simulink model "Simulacion_stepper_2024a"  (R2024a)
settings: Solver=ode4  StartTime=0.0  StopTime=Time_simulation  FixedStep=1/frecuency_simulation  RelTol=1e-3
InitFcn:
  | %%InitFcn();
StopFcn:
  | %%FinishFcn
model workspace (MAT data in the model file):
  Ts_stepper = 0.001
values from neighbouring files (symbols this model uses):
  B = motor_params.B_internal    [bode.m]    (also in current_observer.m = 0.0005; discretizacion.m = [ 1/L, 0; ekf_4_estados.m = params.B; obs_ctrl_back_emf_ext.m = [1/L 0)
  B0 = 3*wn_w - BJ_hat    [Barrido_B.m]    (also in Barrido_J.m; InitFcn.m = 449.962302294)
  B1 = 3*wn_w^2 - B0*BJ_hat    [Barrido_B.m]    (also in Barrido_J.m; InitFcn.m = 64448.3670019)
  B2 = -(J_var/P)*(wn_w^3)    [Barrido_B.m]    (also in Barrido_J.m; InitFcn.m = -0.364323750994)
  B_internal = 1e-4    (= 0.0001)    [InitFcn.m]
  B_var = B_internal* B_factors(k)    [Barrido_B.m]    (also in Barrido_J.m = B_real; InitFcn.m = 0.0001)
  frecuency_simulation = 10e3    (= 10000)    [InitFcn.m]
  I_nom = 1    [InitFcn.m]    (also in salient_motor.m)
  J = motor_params.J_internal    [bode.m]    (also in current_observer.m = 0.008; ekf_4_estados.m = params.J; obs_ctrl_back_emf_ext.m = 0.008; obs_y_contrl_back_emd.m = 0.008)
  J_internal = 4.7/1000000    (= 4.7e-06)    [InitFcn.m]
  J_var = J_real    [Barrido_B.m]    (also in Barrido_J.m = J_internal * J_factors(k); InitFcn.m = 4.7e-06)
  Ke = Kt    [InitFcn.m]    (also in current_observer.m = 0.0055; ekf_4_estados.m = params.Ke; observer.m = Pvec(3); salient_motor.m = 0.0066)
  Ki_d = wd_d*R    (= 3926.99081699)    [InitFcn.m]    (also in bode.m = PI_dq_params.Ki_d_salient)
  Ki_d_salient = wd_d^2*Ld    (= 21491.0635834)    [InitFcn.m]
  Ki_q = wd_q*R    (= 3926.99081699)    [InitFcn.m]    (also in bode.m = PI_dq_params.Ki_q_salient)
  Ki_q_salient = wd_q^2*Lq    (= 7846.33549887)    [InitFcn.m]
  Ki_w = (wn_w^2)*J_var/Kt    [Barrido_B.m]    (also in Barrido_J.m; InitFcn.m; bode.m = PI_MTPA_params.Ki_w)
  Kp_d = wd_d*L    (= 9.42477796077)    [InitFcn.m]    (also in bode.m = PI_dq_params.Kp_d_salient)
  Kp_d_salient = 2*shi_d*wd_d*Ld -R    (= 16.845833313)    [InitFcn.m]
  Kp_q = wd_q*L    (= 9.42477796077)    [InitFcn.m]    (also in bode.m = PI_dq_params.Kp_q_salient)
  Kp_q_salient = 2*shi_q*wd_q*Lq-R    (= 4.56311709936)    [InitFcn.m]
  Kp_w = (2*shi_w*wn_w*J_var)/Kt    [Barrido_B.m]    (also in Barrido_J.m; InitFcn.m; bode.m = PI_MTPA_params.Kp_w)
  Kt = Thold / (sqrt(2) * I_nom)    [InitFcn.m]    (also in current_observer.m = 0.275; ekf_4_estados.m = params.Kt; frecuencia_max.m = 0.33; observer.m = Pvec(4))
  L = 6/1000    (= 0.006)    [InitFcn.m]    (also in current_observer.m = place(A', C', 10*eig(A)).'; desfase.m = lags(k); discretizacion.m = 0.01; frecuencia_max.m)
  Ld = L0 + L2    [Copy_of_PMSM_salient.m]    (also in InitFcn.m = 0.00871; bode.m = motor_params.Ld; ekf_4_estados.m = params.Ld; salient_motor.m = 0.00871)
  Lq = L0 - L2    [Copy_of_PMSM_salient.m]    (also in InitFcn.m = 0.00318; bode.m = motor_params.Lq; ekf_4_estados.m = params.Lq; salient_motor.m = 0.00318)
  N_steps = 360/Step_angle    (= 200)    [InitFcn.m]
  P = N_teeths/2    (= 50)    [InitFcn.m]    (also in bode.m = motor_params.P; ekf_4_estados.m = P_pred; frecuencia_max.m; salient_motor.m)
  Phi = pi/2    (= 1.57079632679)    [InitFcn.m]    (also in ekf_4_estados.m = eye(4) + Ts_eff*A)
  Psi = Kt/P    [InitFcn.m]    (also in bode.m = motor_params.Ke; salient_motor.m = 0.0066)
  R = 2.5    [InitFcn.m]    (also in bode.m = motor_params.R; current_observer.m = 3.4; discretizacion.m = 3.4; ekf_4_estados.m = params.R)
  sample_time = 1/frecuency_simulation    (= 0.0001)    [InitFcn.m]
  Tdm = 18/1000    (= 0.018)    [InitFcn.m]    (also in salient_motor.m)
  Ts_current = 1/f_current    (= 0.0001)    [InitFcn.m]
  Ts_DO = Ts_Wm    (= 0.0001)    [InitFcn.m]
  Ts_ekf = 1/f_ekf    (= 0.0001)    [InitFcn.m]
  Ts_Wm = Ts_current    (= 0.0001)    [InitFcn.m]
  Vdc = 12    [InitFcn.m]    (also in frecuencia_max.m)
undefined symbols (not defined in the file or in its folder): DiscIntNeverNeededParam
libraries: fl_lib x27, nesl_utility x19, spsMosfetLib x16, simulink x8, eeTransforms x4, spsDCVoltageSourceLib x4, spsVoltageMeasurementLib x4, ee_lib x3, slexportprevious_tp74def212_4eb8_4616_a2bc_f4e795655e99 x1, spsTriangleGeneratorLib x1, spspowerguiLib x1
(part 3 of 4)

== system Simulacion_stepper_2024a/Triggered Subsystem8 ==
  Wm_ref : Inport
  Wm : Inport  Port=2
  Tl_Tdm : Inport  Port=3
  function : TriggerPort  TriggerType=function-call  VariantControl=(inherit)  SampleTime=1/100
  C/C++ Code Block : S-Function  Commented=on  FunctionName=PI_dq  SFunctionModules=PI_dq_wrapper.c  SFunctionDeploymentMode=off  EnableBusSupport=off  mask(S-Function Builder){}
      mask help: Simulink:masks:SFunctionBuilder_MD
      mask init: same as Simulacion_stepper_2024a/Triggered Subsystem1/C/C++ Code Block1
      settings: CopyFcn=set_param(gcbh,'LinkStatus','none')  OpenFcn=sfunctionwizard(gcbh)
      mask Display:
      | plot(val(:,1),val(:,2))
      | disp(sys)
      | port_label('input',1,sprintf('%s', 'Ia'),'interpreter','tex')
      | port_label('input',2,sprintf('%s', 'Ib'),'interpreter','tex')
      | port_label('input',3,sprintf('%s', 'Wm\_ref'),'interpreter','tex')
      | port_label('input',4,sprintf('%s', 'Wm\_ext'),'interpreter','tex')
      | port_label('input',5,sprintf('%s', 'Kp\_current'),'interpreter','tex')
      | port_label('input',6,sprintf('%s', 'Ki\_current'),'interpreter','tex')
      | port_label('input',7,sprintf('%s', 'Kd\_current'),'interpreter','tex')
      | port_label('input',8,sprintf('%s', 'sample\_time\_ext'),'interpreter','tex')
      | port_label('input',9,sprintf('%s', 'Vdc\_ext'),'interpreter','tex')
      | port_label('input',10,sprintf('%s', 'R\_ext'),'interpreter','tex')
      | port_label('input',11,sprintf('%s', 'Ld\_ext'),'interpreter','tex')
      | port_label('input',12,sprintf('%s', 'Lq\_ext'),'interpreter','tex')
      | port_label('input',13,sprintf('%s', 'Ke\_ext'),'interpreter','tex')
      | port_label('input',14,sprintf('%s', 'Theta\_ext'),'interpreter','tex')
      | port_label('input',15,sprintf('%s', 'Kp\_wm'),'interpreter','tex')
      | port_label('input',16,sprintf('%s', 'Ki\_wm'),'interpreter','tex')
      | port_label('input',17,sprintf('%s', 'Tl\_Tdm'),'interpreter','tex')
      | port_label('input',18,sprintf('%s', 'B'),'interpreter','tex')
      | port_label('input',19,sprintf('%s', 'Kt\_ext'),'interpreter','tex')
      | port_label('output',1,sprintf('%s', 'Ud'),'interpreter','tex')
      | port_label('output',2,sprintf('%s', 'Uq'),'interpreter','tex')
      | port_label('output',3,sprintf('%s', 'Id'),'interpreter','tex')
      | port_label('output',4,sprintf('%s', 'Iq'),'interpreter','tex')
      | port_label('output',5,sprintf('%s', 'Iq\_ref\_aux'),'interpreter','tex')
  Constant : Constant  Value=B_var  OutDataTypeStr=double
  Constant1 : Constant  Value=Kp_w  OutDataTypeStr=double
  Constant11 : Constant  Value=Ki_w  OutDataTypeStr=double
  Constant12 : Constant  Value=Kt  OutDataTypeStr=double
  Constant2 : Constant  Value=I_nom  OutDataTypeStr=double
  Constant3 : Constant  Value=Ts_Wm  OutDataTypeStr=double
  MATLAB Function : MATLAB Function  TreatAsAtomicUnit=on
  Iq_ref : Outport
  wires:
  MATLAB Function/1(Iq_ref) -> Iq_ref/1
  Wm_ref/1 -> MATLAB Function/1(Wm_ref)
  Wm/1 -> MATLAB Function/2(Wm)
  Constant12/1 -> MATLAB Function/8(Kt)
  Constant/1 -> MATLAB Function/7(B)
  Tl_Tdm/1 -> MATLAB Function/6(Tl_tdm)
  Constant1/1 -> MATLAB Function/4(Kp_w)
  Constant11/1 -> MATLAB Function/5(Ki_w)
  Constant3/1 -> MATLAB Function/3(Ts)
  Constant2/1 -> MATLAB Function/9(Imax)

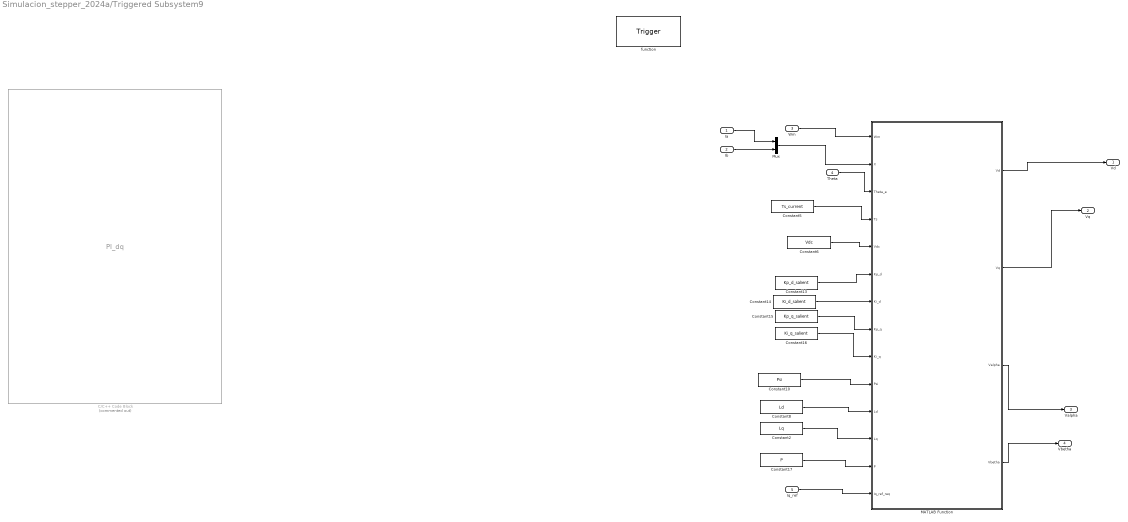
== system Simulacion_stepper_2024a/Triggered Subsystem9 ==
  Ia : Inport
  Ib : Inport  Port=2
  Wm : Inport  Port=3
  Theta : Inport  Port=4
  Iq_ref : Inport  Port=5
  function : TriggerPort  TriggerType=function-call  VariantControl=(inherit)  SampleTime=1/100
  C/C++ Code Block : S-Function  Commented=on  FunctionName=PI_dq  SFunctionModules=PI_dq_wrapper.c  SFunctionDeploymentMode=off  EnableBusSupport=off  mask(S-Function Builder){}
      mask help: Simulink:masks:SFunctionBuilder_MD
      mask init: same as Simulacion_stepper_2024a/Triggered Subsystem1/C/C++ Code Block1
      settings: CopyFcn=set_param(gcbh,'LinkStatus','none')  OpenFcn=sfunctionwizard(gcbh)
      mask Display:
      | plot(val(:,1),val(:,2))
      | disp(sys)
      | port_label('input',1,sprintf('%s', 'Ia'),'interpreter','tex')
      | port_label('input',2,sprintf('%s', 'Ib'),'interpreter','tex')
      | port_label('input',3,sprintf('%s', 'Wm\_ref'),'interpreter','tex')
      | port_label('input',4,sprintf('%s', 'Wm\_ext'),'interpreter','tex')
      | port_label('input',5,sprintf('%s', 'Kp\_current'),'interpreter','tex')
      | port_label('input',6,sprintf('%s', 'Ki\_current'),'interpreter','tex')
      | port_label('input',7,sprintf('%s', 'Kd\_current'),'interpreter','tex')
      | port_label('input',8,sprintf('%s', 'sample\_time\_ext'),'interpreter','tex')
      | port_label('input',9,sprintf('%s', 'Vdc\_ext'),'interpreter','tex')
      | port_label('input',10,sprintf('%s', 'R\_ext'),'interpreter','tex')
      | port_label('input',11,sprintf('%s', 'Ld\_ext'),'interpreter','tex')
      | port_label('input',12,sprintf('%s', 'Lq\_ext'),'interpreter','tex')
      | port_label('input',13,sprintf('%s', 'Ke\_ext'),'interpreter','tex')
      | port_label('input',14,sprintf('%s', 'Theta\_ext'),'interpreter','tex')
      | port_label('input',15,sprintf('%s', 'Kp\_wm'),'interpreter','tex')
      | port_label('input',16,sprintf('%s', 'Ki\_wm'),'interpreter','tex')
      | port_label('input',17,sprintf('%s', 'Tl\_Tdm'),'interpreter','tex')
      | port_label('input',18,sprintf('%s', 'B'),'interpreter','tex')
      | port_label('input',19,sprintf('%s', 'Kt\_ext'),'interpreter','tex')
      | port_label('output',1,sprintf('%s', 'Ud'),'interpreter','tex')
      | port_label('output',2,sprintf('%s', 'Uq'),'interpreter','tex')
      | port_label('output',3,sprintf('%s', 'Id'),'interpreter','tex')
      | port_label('output',4,sprintf('%s', 'Iq'),'interpreter','tex')
      | port_label('output',5,sprintf('%s', 'Iq\_ref\_aux'),'interpreter','tex')
  Constant10 : Constant  Value=Psi  OutDataTypeStr=double
  Constant13 : Constant  Value=Kp_d_salient  OutDataTypeStr=double
  Constant14 : Constant  Value=Ki_d_salient  OutDataTypeStr=double
  Constant15 : Constant  Value=Kp_q_salient  OutDataTypeStr=double
  Constant16 : Constant  Value=Ki_q_salient  OutDataTypeStr=double
  Constant17 : Constant  Value=P  OutDataTypeStr=double
  Constant2 : Constant  Value=Lq  OutDataTypeStr=double
  Constant5 : Constant  Value=Ts_current  OutDataTypeStr=double
  Constant6 : Constant  Value=Vdc  OutDataTypeStr=double
  Constant8 : Constant  Value=Ld  OutDataTypeStr=double
  MATLAB Function : MATLAB Function  TreatAsAtomicUnit=on
  Mux : Mux  Inputs=2
  Vd : Outport
  Vq : Outport  Port=2
  Valpha : Outport  Port=3
  Vbetha : Outport  Port=4
  wires:
  MATLAB Function/1(Vd) -> Vd/1
  Wm/1 -> MATLAB Function/1(Wm)
  Ia/1 -> Mux/1
  Ib/1 -> Mux/2
  Mux/1 -> MATLAB Function/2(X)
  Theta/1 -> MATLAB Function/3(Theta_e)
  Constant5/1 -> MATLAB Function/4(Ts)
  Constant6/1 -> MATLAB Function/5(Vdc)
  Constant13/1 -> MATLAB Function/6(Kp_d)
  Constant14/1 -> MATLAB Function/7(Ki_d)
  Constant15/1 -> MATLAB Function/8(Kp_q)
  Constant16/1 -> MATLAB Function/9(Ki_q)
  Constant10/1 -> MATLAB Function/10(Psi)
  Constant8/1 -> MATLAB Function/11(Ld)
  Constant17/1 -> MATLAB Function/13(P)
  Constant2/1 -> MATLAB Function/12(Lq)
  MATLAB Function/2(Vq) -> Vq/1
  Iq_ref/1 -> MATLAB Function/14(Iq_ref_req)
  MATLAB Function/3(Valpha) -> Valpha/1
  MATLAB Function/4(Vbetha) -> Vbetha/1

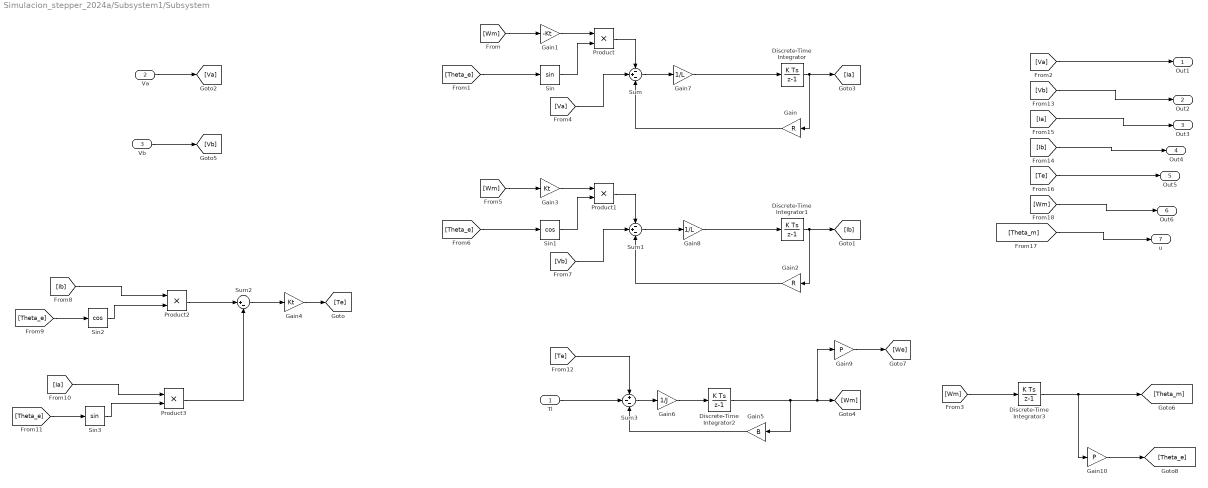
== system Simulacion_stepper_2024a/Subsystem1/Subsystem ==
  Tl : Inport
  Va : Inport  Port=2
  Vb : Inport  Port=3
  Discrete-Time Integrator{,1..3} (4 alike) : DiscreteIntegrator  SampleTime=sample_time  ICPrevOutput=DiscIntNeverNeededParam  ICPrevScaledInput=DiscIntNeverNeededParam
  Gain : Gain  Gain=R
  Gain1 : Gain  Gain=-Kt
  Gain10 : Gain  Gain=P
  Gain2 : Gain  Gain=R
  Gain3 : Gain  Gain=Kt
  Gain4 : Gain  Gain=Kt
  Gain5 : Gain  Gain=B
  Gain6 : Gain  Gain=1/J
  Gain7 : Gain  Gain=1/L
  Gain8 : Gain  Gain=1/L
  Gain9 : Gain  Gain=P
  Product{,1..3} (4 alike) : Product
  Sin : Trigonometry
  Sin1 : Trigonometry  Operator=cos
  Sin2 : Trigonometry  Operator=cos
  Sin3 : Trigonometry
  Sum : Sum  Inputs=-+-
  Sum1 : Sum  Inputs=-+-
  Sum2 : Sum  Inputs=|+-
  Sum3 : Sum  Inputs=+--
  Out1 : Outport
  Out2 : Outport  Port=2
  Out3 : Outport  Port=3
  Out4 : Outport  Port=4
  Out5 : Outport  Port=5
  Out6 : Outport  Port=6
  u : Outport  Port=7
  wires:
  Discrete-Time Integrator/1 -> [Ia], Gain/1
  Discrete-Time Integrator2/1 -> Gain5/1, Gain9/1, [Wm]
  [Wm] -> Discrete-Time Integrator3/1
  [Vb] -> Out2/1
  [Ia] -> Out3/1
  [Ib] -> Out4/1
  [Te] -> Out5/1
  [Wm] -> Out6/1
  [Theta_m] -> u/1
  [Va] -> Out1/1
  Discrete-Time Integrator3/1 -> Gain10/1, [Theta_m]
  Vb/1 -> [Vb]
  Va/1 -> [Va]
  [Wm] -> Gain1/1
  Gain1/1 -> Product/1
  Sin/1 -> Product/2
  [Theta_e] -> Sin/1
  Product/1 -> Sum/1
  [Va] -> Sum/2
  Gain/1 -> Sum/3
  Gain2/1 -> Sum1/3
  [Wm] -> Gain3/1
  [Vb] -> Sum1/2
  [Theta_e] -> Sin1/1
  Gain3/1 -> Product1/1
  Sin1/1 -> Product1/2
  Discrete-Time Integrator1/1 -> [Ib], Gain2/1
  Product1/1 -> Sum1/1
  [Ib] -> Product2/1
  Sin2/1 -> Product2/2
  [Theta_e] -> Sin2/1
  [Ia] -> Product3/1
  [Theta_e] -> Sin3/1
  Sin3/1 -> Product3/2
  Product2/1 -> Sum2/1
  Product3/1 -> Sum2/2
  Sum2/1 -> Gain4/1
  Gain4/1 -> [Te]
  [Te] -> Sum3/1
  Tl/1 -> Sum3/2
  Gain5/1 -> Sum3/3
  Sum3/1 -> Gain6/1
  Sum/1 -> Gain7/1
  Gain7/1 -> Discrete-Time Integrator/1
  Sum1/1 -> Gain8/1
  Gain8/1 -> Discrete-Time Integrator1/1
  Gain6/1 -> Discrete-Time Integrator2/1
  Gain9/1 -> [We]
  Gain10/1 -> [Theta_e]

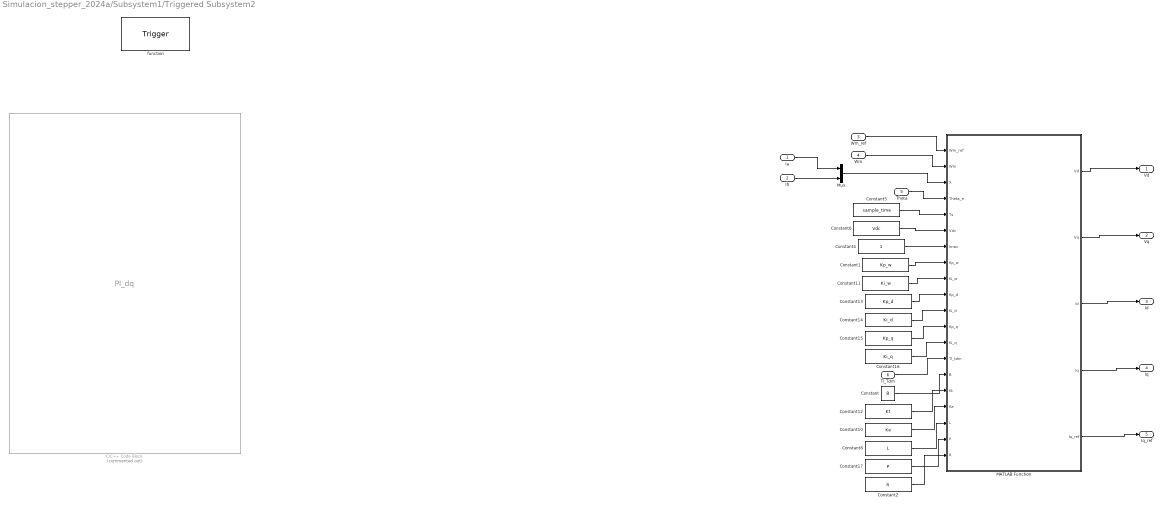
== system Simulacion_stepper_2024a/Subsystem1/Triggered Subsystem2 ==
  Ia : Inport
  Ib : Inport  Port=2
  Wm_ref : Inport  Port=3
  Wm : Inport  Port=4
  Theta : Inport  Port=5
  Tl_Tdm : Inport  Port=6
  function : TriggerPort  TriggerType=function-call  VariantControl=(inherit)  SampleTime=1/100
  C/C++ Code Block : S-Function  Commented=on  FunctionName=PI_dq  SFunctionModules=PI_dq_wrapper.c  SFunctionDeploymentMode=off  EnableBusSupport=off  mask(S-Function Builder){}
      mask help: Simulink:masks:SFunctionBuilder_MD
      mask init: same as Simulacion_stepper_2024a/Triggered Subsystem1/C/C++ Code Block1
      settings: CopyFcn=set_param(gcbh,'LinkStatus','none')  OpenFcn=sfunctionwizard(gcbh)
      mask Display:
      | plot(val(:,1),val(:,2))
      | disp(sys)
      | port_label('input',1,sprintf('%s', 'Ia'),'interpreter','tex')
      | port_label('input',2,sprintf('%s', 'Ib'),'interpreter','tex')
      | port_label('input',3,sprintf('%s', 'Wm\_ref'),'interpreter','tex')
      | port_label('input',4,sprintf('%s', 'Wm\_ext'),'interpreter','tex')
      | port_label('input',5,sprintf('%s', 'Kp\_current'),'interpreter','tex')
      | port_label('input',6,sprintf('%s', 'Ki\_current'),'interpreter','tex')
      | port_label('input',7,sprintf('%s', 'Kd\_current'),'interpreter','tex')
      | port_label('input',8,sprintf('%s', 'sample\_time\_ext'),'interpreter','tex')
      | port_label('input',9,sprintf('%s', 'Vdc\_ext'),'interpreter','tex')
      | port_label('input',10,sprintf('%s', 'R\_ext'),'interpreter','tex')
      | port_label('input',11,sprintf('%s', 'Ld\_ext'),'interpreter','tex')
      | port_label('input',12,sprintf('%s', 'Lq\_ext'),'interpreter','tex')
      | port_label('input',13,sprintf('%s', 'Ke\_ext'),'interpreter','tex')
      | port_label('input',14,sprintf('%s', 'Theta\_ext'),'interpreter','tex')
      | port_label('input',15,sprintf('%s', 'Kp\_wm'),'interpreter','tex')
      | port_label('input',16,sprintf('%s', 'Ki\_wm'),'interpreter','tex')
      | port_label('input',17,sprintf('%s', 'Tl\_Tdm'),'interpreter','tex')
      | port_label('input',18,sprintf('%s', 'B'),'interpreter','tex')
      | port_label('input',19,sprintf('%s', 'Kt\_ext'),'interpreter','tex')
      | port_label('output',1,sprintf('%s', 'Ud'),'interpreter','tex')
      | port_label('output',2,sprintf('%s', 'Uq'),'interpreter','tex')
      | port_label('output',3,sprintf('%s', 'Id'),'interpreter','tex')
      | port_label('output',4,sprintf('%s', 'Iq'),'interpreter','tex')
      | port_label('output',5,sprintf('%s', 'Iq\_ref\_aux'),'interpreter','tex')
  Constant : Constant  Value=B  OutDataTypeStr=double
  Constant1 : Constant  Value=Kp_w  OutDataTypeStr=double
  Constant10 : Constant  Value=Ke  OutDataTypeStr=double
  Constant11 : Constant  Value=Ki_w  OutDataTypeStr=double
  Constant12 : Constant  Value=Kt  OutDataTypeStr=double
  Constant13 : Constant  Value=Kp_d  OutDataTypeStr=double
  Constant14 : Constant  Value=Ki_d  OutDataTypeStr=double
  Constant15 : Constant  Value=Kp_q  OutDataTypeStr=double
  Constant16 : Constant  Value=Ki_q  OutDataTypeStr=double
  Constant17 : Constant  Value=P  OutDataTypeStr=double
  Constant2 : Constant  Value=R  OutDataTypeStr=double
  Constant4 : Constant  OutDataTypeStr=double
  Constant5 : Constant  Value=sample_time  OutDataTypeStr=double
  Constant6 : Constant  Value=Vdc  OutDataTypeStr=double
  Constant8 : Constant  Value=L  OutDataTypeStr=double
  MATLAB Function : MATLAB Function  TreatAsAtomicUnit=on
  Mux : Mux  Inputs=2
  Vd : Outport
  Vq : Outport  Port=2
  Id : Outport  Port=3
  Iq : Outport  Port=4
  Iq_ref : Outport  Port=5
  wires:
  MATLAB Function/1(Vd) -> Vd/1
  MATLAB Function/2(Vq) -> Vq/1
  MATLAB Function/3(Id) -> Id/1
  MATLAB Function/4(Iq) -> Iq/1
  MATLAB Function/5(Iq_ref) -> Iq_ref/1
  Wm_ref/1 -> MATLAB Function/1(Wm_ref)
  Wm/1 -> MATLAB Function/2(Wm)
  Ia/1 -> Mux/1
  Ib/1 -> Mux/2
  Mux/1 -> MATLAB Function/3(X)
  Theta/1 -> MATLAB Function/4(Theta_e)
  Constant5/1 -> MATLAB Function/5(Ts)
  Constant6/1 -> MATLAB Function/6(Vdc)
  Constant12/1 -> MATLAB Function/16(Kt)
  Constant/1 -> MATLAB Function/15(B)
  Tl_Tdm/1 -> MATLAB Function/14(Tl_tdm)
  Constant1/1 -> MATLAB Function/8(Kp_w)
  Constant11/1 -> MATLAB Function/9(Ki_w)
  Constant13/1 -> MATLAB Function/10(Kp_d)
  Constant14/1 -> MATLAB Function/11(Ki_d)
  Constant15/1 -> MATLAB Function/12(Kp_q)
  Constant16/1 -> MATLAB Function/13(Ki_q)
  Constant10/1 -> MATLAB Function/17(Ke)
  Constant8/1 -> MATLAB Function/18(L)
  Constant17/1 -> MATLAB Function/19(P)
  Constant4/1 -> MATLAB Function/7(Imax)
  Constant2/1 -> MATLAB Function/20(R)

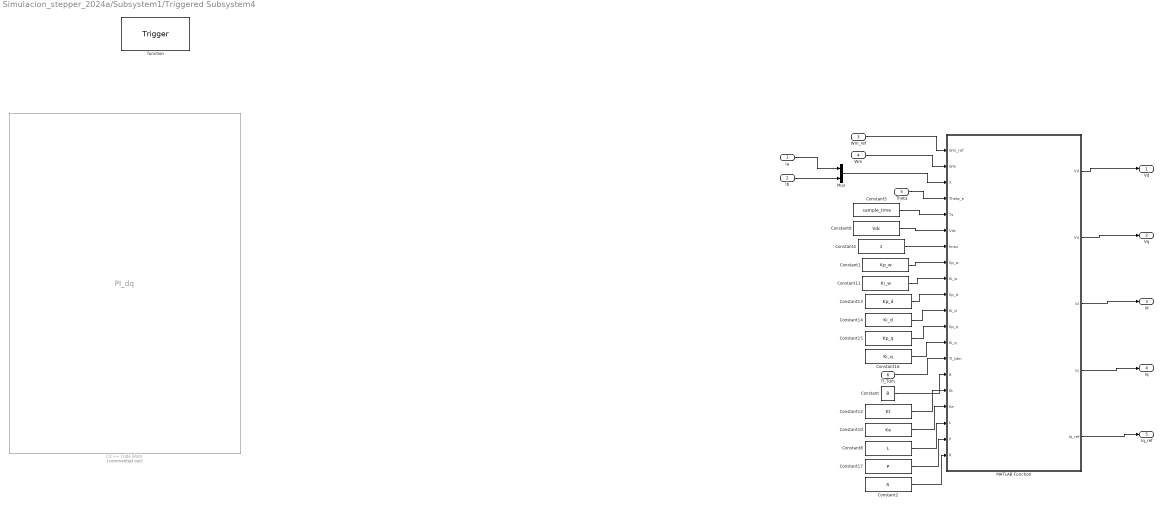
== system Simulacion_stepper_2024a/Subsystem1/Triggered Subsystem4 ==
  Ia : Inport
  Ib : Inport  Port=2
  Wm_ref : Inport  Port=3
  Wm : Inport  Port=4
  Theta : Inport  Port=5
  Tl_Tdm : Inport  Port=6
  function : TriggerPort  TriggerType=function-call  VariantControl=(inherit)  SampleTime=1/100
  C/C++ Code Block : S-Function  Commented=on  FunctionName=PI_dq  SFunctionModules=PI_dq_wrapper.c  SFunctionDeploymentMode=off  EnableBusSupport=off  mask(S-Function Builder){}
      mask help: Simulink:masks:SFunctionBuilder_MD
      mask init: same as Simulacion_stepper_2024a/Triggered Subsystem1/C/C++ Code Block1
      settings: CopyFcn=set_param(gcbh,'LinkStatus','none')  OpenFcn=sfunctionwizard(gcbh)
      mask Display:
      | plot(val(:,1),val(:,2))
      | disp(sys)
      | port_label('input',1,sprintf('%s', 'Ia'),'interpreter','tex')
      | port_label('input',2,sprintf('%s', 'Ib'),'interpreter','tex')
      | port_label('input',3,sprintf('%s', 'Wm\_ref'),'interpreter','tex')
      | port_label('input',4,sprintf('%s', 'Wm\_ext'),'interpreter','tex')
      | port_label('input',5,sprintf('%s', 'Kp\_current'),'interpreter','tex')
      | port_label('input',6,sprintf('%s', 'Ki\_current'),'interpreter','tex')
      | port_label('input',7,sprintf('%s', 'Kd\_current'),'interpreter','tex')
      | port_label('input',8,sprintf('%s', 'sample\_time\_ext'),'interpreter','tex')
      | port_label('input',9,sprintf('%s', 'Vdc\_ext'),'interpreter','tex')
      | port_label('input',10,sprintf('%s', 'R\_ext'),'interpreter','tex')
      | port_label('input',11,sprintf('%s', 'Ld\_ext'),'interpreter','tex')
      | port_label('input',12,sprintf('%s', 'Lq\_ext'),'interpreter','tex')
      | port_label('input',13,sprintf('%s', 'Ke\_ext'),'interpreter','tex')
      | port_label('input',14,sprintf('%s', 'Theta\_ext'),'interpreter','tex')
      | port_label('input',15,sprintf('%s', 'Kp\_wm'),'interpreter','tex')
      | port_label('input',16,sprintf('%s', 'Ki\_wm'),'interpreter','tex')
      | port_label('input',17,sprintf('%s', 'Tl\_Tdm'),'interpreter','tex')
      | port_label('input',18,sprintf('%s', 'B'),'interpreter','tex')
      | port_label('input',19,sprintf('%s', 'Kt\_ext'),'interpreter','tex')
      | port_label('output',1,sprintf('%s', 'Ud'),'interpreter','tex')
      | port_label('output',2,sprintf('%s', 'Uq'),'interpreter','tex')
      | port_label('output',3,sprintf('%s', 'Id'),'interpreter','tex')
      | port_label('output',4,sprintf('%s', 'Iq'),'interpreter','tex')
      | port_label('output',5,sprintf('%s', 'Iq\_ref\_aux'),'interpreter','tex')
  Constant : Constant  Value=B  OutDataTypeStr=double
  Constant1 : Constant  Value=Kp_w  OutDataTypeStr=double
  Constant10 : Constant  Value=Ke  OutDataTypeStr=double
  Constant11 : Constant  Value=Ki_w  OutDataTypeStr=double
  Constant12 : Constant  Value=Kt  OutDataTypeStr=double
  Constant13 : Constant  Value=Kp_d  OutDataTypeStr=double
  Constant14 : Constant  Value=Ki_d  OutDataTypeStr=double
  Constant15 : Constant  Value=Kp_q  OutDataTypeStr=double
  Constant16 : Constant  Value=Ki_q  OutDataTypeStr=double
  Constant17 : Constant  Value=P  OutDataTypeStr=double
  Constant2 : Constant  Value=R  OutDataTypeStr=double
  Constant4 : Constant  OutDataTypeStr=double
  Constant5 : Constant  Value=sample_time  OutDataTypeStr=double
  Constant6 : Constant  Value=Vdc  OutDataTypeStr=double
  Constant8 : Constant  Value=L  OutDataTypeStr=double
  MATLAB Function : MATLAB Function  TreatAsAtomicUnit=on
  Mux : Mux  Inputs=2
  Vd : Outport
  Vq : Outport  Port=2
  Id : Outport  Port=3
  Iq : Outport  Port=4
  Iq_ref : Outport  Port=5
  wires:
  MATLAB Function/1(Vd) -> Vd/1
  MATLAB Function/2(Vq) -> Vq/1
  MATLAB Function/3(Id) -> Id/1
  MATLAB Function/4(Iq) -> Iq/1
  MATLAB Function/5(Iq_ref) -> Iq_ref/1
  Wm_ref/1 -> MATLAB Function/1(Wm_ref)
  Wm/1 -> MATLAB Function/2(Wm)
  Ia/1 -> Mux/1
  Ib/1 -> Mux/2
  Mux/1 -> MATLAB Function/3(X)
  Theta/1 -> MATLAB Function/4(Theta_e)
  Constant5/1 -> MATLAB Function/5(Ts)
  Constant6/1 -> MATLAB Function/6(Vdc)
  Constant12/1 -> MATLAB Function/16(Kt)
  Constant/1 -> MATLAB Function/15(B)
  Tl_Tdm/1 -> MATLAB Function/14(Tl_tdm)
  Constant1/1 -> MATLAB Function/8(Kp_w)
  Constant11/1 -> MATLAB Function/9(Ki_w)
  Constant13/1 -> MATLAB Function/10(Kp_d)
  Constant14/1 -> MATLAB Function/11(Ki_d)
  Constant15/1 -> MATLAB Function/12(Kp_q)
  Constant16/1 -> MATLAB Function/13(Ki_q)
  Constant10/1 -> MATLAB Function/17(Ke)
  Constant8/1 -> MATLAB Function/18(L)
  Constant17/1 -> MATLAB Function/19(P)
  Constant4/1 -> MATLAB Function/7(Imax)
  Constant2/1 -> MATLAB Function/20(R)

== matlab function Simulacion_stepper_2024a/Triggered Subsystem1/MATLAB Function1 ==
  data: U input; x_corr output; X input; Ts input; Kt input; R input; J input; L input; Nr input; B input; Ke input
function x_corr = ekf_5var(U,X,Ts,Kt,R,J,L,Nr,B,Ke)
persistent x_hat P x_pred
%%  x_hat son los estados predichos
%%  x_corr es la salida corregida
%%  P_pre ó Sum_less es la covarianza predicha
%%  P ó sum_more es la covarianza
%%  Rk ó sum_v es la covarianza de incertidumbre del sensor




 %%Iniciamos calculando X_hat[k-1]
 if isempty(x_hat)
     x_hat = zeros(5,1);
     P = diag([1e-4 1e-4 1e-6 1e-10 1e-4]);
     x_corr = zeros(5,1);
     x_pred = zeros(5,1);


 end

Qk = diag([1e-4 1e-4 1e-4 1e-10 1e-6]);
Rk = diag([5e-4 5e-4]);   % ruido de medición

%%1A
%%Predicción
Ia = x_hat(1);
Ib = x_hat(2);
Wm = x_hat(3);
Th_m = x_hat(4);
Tx = x_hat(5);

Th_e = Nr*Th_m;
S = sin(Th_e);
C = cos(Th_e);

Va = U(1);
Vb = U(2);

dx = zeros(5,1);
dx(1) = (Va - R*Ia + Ke*Wm*S)/L;
dx(2) = (Vb - R*Ib - Ke*Wm*C)/L;
dx(3) = (Kt*(Ib*C-Ia*S) -Tx)/J;
dx(4) = Wm;
dx(5) = 0;
x_pred = x_hat + Ts*dx;
x_pred(4) = wrap_2pi(x_pred(4));

%%Calculamos el jacobiano
RL = R/L;
uno = Ke*S;
dos = Ke*C;

A = [-RL 0   (uno/L) (dos*Nr*Wm/L) 0;
 0  -RL   -dos/L    uno*Nr*Wm/L  0;
 -uno/J dos/J -1/J -Kt*Nr*(Ia*C+Ib*S)/J -1/J;
 0 0 1 0 0;
 0 0 0 0 0];

A_hat = eye(5) + Ts*A;
A_hat_T = transpose(A_hat);

%%1B COVARIANZA PREDICHA
P_pred = A_hat * P * A_hat_T + Qk; 


%%1C PREDECIMOS LA SALIDA DEL SISTEMA
Ck = [1 0 0 0 0;
      0 1 0 0 0];
Ck_T = transpose(Ck);
y_pred = Ck*x_pred;

%%2A calculamos la matriz Lk
%%Lk = P_pred *Ck_T * inv(Ck*P_pred*Ck_T + sum_v)
Sk = Ck*P_pred*Ck_T + Rk;
Lk = P_pred * Ck_T /Sk;

%%2B Actualizamos los estados estados corregidos en función de L


y_meas = [X(1);X(2)];

innov = y_meas - y_pred;
x_corr = x_pred + Lk*(innov);
x_corr(4) = wrap_2pi(x_corr(4));
%%actualizamos la covarianza y guardamos el estado
x_hat = x_corr;
Lk_T = transpose(Lk);
P = P_pred - Lk*Sk*Lk_T;
P_T = transpose(P);
P = 0.5 * (P + P_T);

== matlab function Simulacion_stepper_2024a/MATLAB Function4 ==
  data: u input; y output
function y = fcn(u)

y = wrap_2pi(u);

== matlab function Simulacion_stepper_2024a/Triggered Subsystem1/MATLAB Function2 ==
  data: U input size=2; x_corr output; Y input size=2; Ts input; Kt input; R input; J input; L input; Nr input; B input
function x_corr = SPKF_4var(U,Y,Ts,Kt,R,J,L,Nr,B)
persistent x_hat P  alpham alphac Qk Rk h
%%  x_hat son los estados predichos
%%  x_corr es la salida corregida
%%  P_pre ó Sum_less es la covarianza predicha
%%  P ó sum_more es la covarianza
%%  Rk ó sum_v es la covarianza de incertidumbre del sensor


Nx = 4; %%Números de estados
Nw = 4; %% Incertidumbres de estado
Ny = 2; %% Incertidumbre de mediciones
Na = Nx+Nw+Ny;


%%Los métodos de sigma-point pueden diferir al utilizar las variables
%%alpha. Existen 2 métodos:

%% Método |    Sigma       |     alpha_m_0      | alpha_m_k         |           alpha_c_0               | alpha_c_k |
%% UKF    | sqrt(L+lambda) |  lambda/(L+Lambda) | 1/(2*(L+Lambda))  | alpha_m_0 + (1-alpha^2 + betha)   | alpha_m_k |
%% CDKF   |    h           |   (h^2 - L)/h^2    |  1/(2*h^2)        | alpha_m_0                         | alpha_m_k |
 %%Iniciamos calculando X_hat[k-1]
 if isempty(x_hat)
    
     %%Utilizamos el CDKF, con h = sqrt(Nxa); 
        x_hat = zeros(Nx,1);
        h =sqrt(Na);
        alpham = ones(2*Na+1,1) * (1/(2*h^2));
        alpham(1) = (h^2 - Na)/(h^2);   % peso del sigma central
        alphac = alpham;             
     %%Valores de covarianza
     P = diag([1e-2 1e-2 1e-6 1e-12 ]);
     Qk = diag([1e-2 1e-2 1e-8 1e-12 ]);
     Rk = [1e-4 0; 0 1e-4];
 end
    
     x_corr = zeros(Nx,1);
     x_pred = zeros(Nx,1);
     x_hat_a = zeros(Na,1);
     X_minus = zeros(Nx,2*Na+1);
     Y_minus = zeros(Ny,2*Na+1);
%%Ciclo de 2*Na+1
%%Aun que deberiamos hacer un ciclo for, en matlab se hace solo asi que no
%%es necesario

%% 1A-I Creamos el vector de estados extendidos
x_hat_a = [x_hat;zeros(Nw,1);zeros(Ny,1)]; 


%% 1A-II Conseguimos el factor de cholesky


%%Creamos la matriz de covarianza extendidas, el cual es de la forma
%%             [P   0    0]
%%     P_a =   [0   Qk   0]
%%             [0   0   Rk]

P_a = blkdiag(P,Qk,Rk);
Sa = chol(P_a,"lower");

%% 1A-III generamos los sigma points
%% Queda de la forma [x_hat_a, x_hat_a + h*S,x_hat_a - h*S] (Por eso es 2*Nxa+1 = N)
%% Al usar x_a x_a(:,ones(1,Na)) creamos una matriz de la forma [x_a,x_a...x_a], que es de tamaño (Na)x(2*Na+1)
%% Posteriormente, se le suma un vector de [0,+h*S,-h*S]
%% Cómo S es del tamaño (Nxa)x(Nxa), el total es de (2*Na+1 = N)
X =  x_hat_a(:,ones(1,2*Na+1)) + h*[zeros(Na,1), Sa, -Sa];

%% 1A-IV Calculamos las ecuaciones de estado
Va = U(1);
Vb = U(2);


for k=1:2*Na+1

  % --- separar estado, ruido de proceso y ruido de medición ---


xk = X(1:Nx,k);                     % [Ia; Ib; Wm; Th_m]
wk = X(Nx+1 : Nx+Nw,k);             % ruido de proceso (4x1)
vk = X(Nx+Nw+1 : end,k);            % ruido de medición (2x1)    

Ia = xk(1);
Ib = xk(2);
Wm = xk(3);
Th_m = xk(4);

Th_e = Nr*Th_m;
S = sin(Th_e);
C = cos(Th_e);


dx1 = (Va - R*Ia + Kt*Wm*S)/L;
dx2 = (Vb - R*Ib - Kt*Wm*C)/L;
dx3 = (Kt*(Ib*C-Ia*S)-B*Wm)/J;
dx4 = Wm;

%Calculamos el paso siguiente mediante euler
%% X_minus corresponde a la matriz que contiene todos los sigma-points distribuidos en los estados del sistema no-extendido (Nx)x(Na)
X_minus(1,k) = Ia + Ts*dx1+ wk(1);
X_minus(2,k) = Ib + Ts*dx2 + wk(2);
X_minus(3,k) = Wm + Ts*dx3 + wk(3);
X_minus(4,k) = Th_m + Ts*dx4 + wk(4);
%%X_minus(4,k) = wrap_2pi(X_minus(4,k));

Y_minus(1,k) = X_minus(1,k) + vk(1);
Y_minus(2,k) = X_minus(2,k) + vk(2);

end
%% 1B Reconstrucción de la media
%% Esta matriz contiene la media de todos los estados. (Nx)x(1)
x_pred = X_minus*alpham;
y_pred = Y_minus*alpham;
%%  Reconstrucción de la covarianza

%% Acá lo que hacemos es copiar la media N veces, para poder realizar la resta.
%%Pero realmente debería ser un for de [Xs(i,k)= X_minus(i,k) - x_pred(i)],
%%dónde K es cada variable de estado (Nx)
%% Xs es una matriz de desviación respecto a la media. Es necesario para construir la covarianza P
Xs = X_minus - x_pred(:,ones([1 2*Na+1])); 
Ys = Y_minus - y_pred(:,ones([1 2*Na+1]));

Xs_T = transpose(Xs);
Ys_T = transpose(Ys);
%%Calculamos la matriz de covarianza, pero hay que considerar que como
%%diag(alphac) es una matriz llena de diagonales, uno puede reducir la
%%cantidad de cómputo.
P_pred = Xs*diag(alphac)*Xs_T;
Pyy = Ys* diag(alphac)* Ys_T;
Pxy = Xs*diag(alphac)*Ys_T;
Lk = Pxy/Pyy;
Lk_T = transpose(Lk);
%% 2B Leemos la medición y actualizamos
x_corr = x_pred + Lk*(Y - y_pred);
x_corr(4) = wrap_2pi(x_corr(4));
%%Guardamos los valores de x_hat para mantenerlos
x_hat = x_corr; 
%% 2C Actualizamos la covarianza
P = P_pred - Lk*Pyy*Lk_T;
P_T = transpose(P);
P = 0.5 * (P + P_T);

== matlab function Simulacion_stepper_2024a/Triggered Subsystem1/MATLAB Function3 ==
  data: U input size=2; x_corr output; Y input size=2; Ts input; Kt input; R input; J input; L input; Nr input; B input
function x_corr = SPKF_5var(U,Y,Ts,Kt,R,J,L,Nr,B)
persistent x_hat P x_pred alpham alphac Qk Rk h
%%  x_hat son los estados predichos
%%  x_corr es la salida corregida
%%  P_pre ó Sum_less es la covarianza predicha
%%  P ó sum_more es la covarianza
%%  Rk ó sum_v es la covarianza de incertidumbre del sensor


Nx = 5; %%Números de estados
Nw = 5; %% Incertidumbres de estado
Ny = 2; %% Incertidumbre de mediciones
Na = Nx+Nw+Ny;


%%Los métodos de sigma-point pueden diferir al utilizar las variables
%%alpha. Existen 2 métodos:

%% Método |    Sigma       |     alpha_m_0      | alpha_m_k         |           alpha_c_0               | alpha_c_k |
%% UKF    | sqrt(L+lambda) |  lambda/(L+Lambda) | 1/(2*(L+Lambda))  | alpha_m_0 + (1-alpha^2 + betha)   | alpha_m_k |
%% CDKF   |    h           |   (h^2 - L)/h^2    |  1/(2*h^2)        | alpha_m_0                         | alpha_m_k |
 %%Iniciamos calculando X_hat[k-1]
 if isempty(x_hat)
    
     %%Utilizamos el CDKF, con h = sqrt(Nxa); 
        x_hat = zeros(Nx,1);
        h =sqrt(Na);
        alpham = ones(2*Na+1,1) * (1/(2*h^2));
        alpham(1) = (h^2 - Na)/(h^2);   % peso del sigma central
        alphac = alpham;             
     %%Valores de covarianza
     P = diag([1e-2 1e-2 1e-4 1e-8 1e-12]);
     Qk = diag([1e-2 1e-2 1e-6 1e-8 1e-12]);
     Rk = [1e-4 0; 0 1e-4];
 end
    
     x_corr = zeros(Nx,1);
     x_pred = zeros(Nx,1);
     x_hat_a = zeros(Na,1);
     X_minus = zeros(Nx,2*Na+1);
     Y_minus = zeros(Ny,2*Na+1);
%%Ciclo de 2*Na+1
%%Aun que deberiamos hacer un ciclo for, en matlab se hace solo asi que no
%%es necesario

%% 1A-I Creamos el vector de estados extendidos
x_hat_a = [x_hat;zeros(Nw,1);zeros(Ny,1)]; 


%% 1A-II Conseguimos el factor de cholesky


%%Creamos la matriz de covarianza extendidas, el cual es de la forma
%%             [P   0    0]
%%     P_a =   [0   Qk   0]
%%             [0   0   Rk]

P_a = blkdiag(P,Qk,Rk);
Sa = chol(P_a,"lower");

%% 1A-III generamos los sigma points
%% Queda de la forma [x_hat_a, x_hat_a + h*S,x_hat_a - h*S] (Por eso es 2*Nxa+1 = N)
%% Al usar x_a x_a(:,ones(1,Na)) creamos una matriz de la forma [x_a,x_a...x_a], que es de tamaño (Na)x(2*Na+1)
%% Posteriormente, se le suma un vector de [0,+h*S,-h*S]
%% Cómo S es del tamaño (Nxa)x(Nxa), el total es de (2*Na+1 = N)
X =  x_hat_a(:,ones(1,2*Na+1)) + h*[zeros(Na,1), Sa, -Sa];

%% 1A-IV Calculamos las ecuaciones de estado
Va = U(1);
Vb = U(2);


for k=1:2*Na+1

  % --- separar estado, ruido de proceso y ruido de medición ---


xk = X(1:Nx,k);                     % [Ia; Ib; Wm; Th_m]
wk = X(Nx+1 : Nx+Nw,k);             % ruido de proceso (4x1)
vk = X(Nx+Nw+1 : end,k);            % ruido de medición (2x1)    

Ia = xk(1);
Ib = xk(2);
Wm = xk(3);
Th_m = xk(4);
Tx = xk(5);

Th_e = Nr*Th_m;
S = sin(Th_e);
C = cos(Th_e);


dx1 = (Va - R*Ia + Kt*Wm*S)/L;
dx2 = (Vb - R*Ib - Kt*Wm*C)/L;
dx3 = (Kt*(Ib*C-Ia*S)-B*Wm - Tx)/J;
dx4 = Wm;
dTx = 0;

%Calculamos el paso siguiente mediante euler
%% X_minus corresponde a la matriz que contiene todos los sigma-points distribuidos en los estados del sistema no-extendido (Nx)x(Na)
X_minus(1,k) = Ia + Ts*dx1+ wk(1);
X_minus(2,k) = Ib + Ts*dx2 + wk(2);
X_minus(3,k) = Wm + Ts*dx3 + wk(3);
X_minus(4,k) = Th_m + Ts*dx4 + wk(4);
X_minus(4,k) = wrap_2pi(X_minus(4,k));
X_minus(5,k) = Tx + Ts*dTx + wk(5);

Y_minus(1,k) = X_minus(1,k) + vk(1);
Y_minus(2,k) = X_minus(2,k) + vk(2);

end
%% 1B Reconstrucción de la media
%% Esta matriz contiene la media de todos los estados. (Nx)x(1)
x_pred = X_minus*alpham;
y_pred = Y_minus*alpham;
%%  Reconstrucción de la covarianza

%% Acá lo que hacemos es copiar la media N veces, para poder realizar la resta.
%%Pero realmente debería ser un for de [Xs(i,k)= X_minus(i,k) - x_pred(i)],
%%dónde K es cada variable de estado (Nx)
%% Xs es una matriz de desviación respecto a la media. Es necesario para construir la covarianza P
Xs = X_minus - x_pred(:,ones([1 2*Na+1])); 
Ys = Y_minus - y_pred(:,ones([1 2*Na+1]));

Xs_T = transpose(Xs);
Ys_T = transpose(Ys);
%%Calculamos la matriz de covarianza, pero hay que considerar que como
%%diag(alphac) es una matriz llena de diagonales, uno puede reducir la
%%cantidad de cómputo.
P_pred = Xs*diag(alphac)*Xs_T;
Pyy = Ys* diag(alphac)* Ys_T;
Pxy = Xs*diag(alphac)*Ys_T;
Lk = Pxy/Pyy;
Lk_T = transpose(Lk);
%% 2B Leemos la medición y actualizamos
x_corr = x_pred + Lk*(Y - y_pred);
x_corr(4) = wrap_2pi(x_corr(4));
%%Guardamos los valores de x_hat para mantenerlos
x_hat = x_corr; 
%% 2C Actualizamos la covarianza
P = P_pred - Lk*Pyy*Lk_T;
P_T = transpose(P);
P = 0.5 * (P + P_T);

== matlab function Simulacion_stepper_2024a/Triggered Subsystem3/MATLAB Function1 ==
  data: theta_EKF input; Iq_obs input; Id_obs input; Ld input; Lq input; Ts input; Kt input; np input; J input; theta_hat output; omega_hat output; d_hat output; B input; beta0 input; beta1 input; beta2 input
function [theta_hat, omega_hat, d_hat] = DO_paper( ...
        theta_EKF,Iq_obs,Id_obs,Ld,Lq, Ts, Kt, np, J, B, beta0, beta1, beta2)

% -----------------------------------------------------------
% Disturbance Observer (Linear DO) from Eq. (36) of the paper:
%   "Simultaneous State and Disturbance Estimation for 
%         Sensorless PMSM Control"
%
% Inputs:
%   theta_EKF  = \hatθ_e^E[k] (EKF estimated electrical angle)
%   omega_EKF  = \hatω_e^E[k] (EKF estimated electrical speed)
%   iq         = i_q(k)
%   Ts         = sampling period
%   Kt         = torque constant in dq model (Kτ)
%   np         = pole pairs
%   J          = inertia
%   B          = viscous friction
%   beta0,beta1,beta2 = DO gains
%
% Outputs:
%   theta_hat = \hatθ_e[k]
%   omega_hat = \hatω_e[k]
%   d_hat     = \hat d[k]  (estimated load torque T_L)
% -----------------------------------------------------------

persistent theta omega d

if isempty(theta)
    theta = 0;
    omega = 0;
    d     = 0;
end

%% ============================
%  (1) Error term Eq. (36)
% =============================
% e0 = θ_E^E[k] − θ̂_e[k−1]
e0 = wrap_2pi(theta_EKF - theta);

%% ============================
%  (2) Angle update Eq. (36)
% ============================
theta_hat = theta + Ts*( omega + beta0 * e0 );
theta_hat = wrapTo2Pi(theta_hat);

%% ============================
%  (3) Speed update Eq. (36)
% ============================
omega_hat = omega ...
    + Ts * ( (Kt * Iq_obs + (Ld-Lq)*Id_obs*Iq_obs)/J ...
           - (np/J) * d ...
           - (B/J) * omega ...
           + beta1 * e0 );

%% ============================
%  (4) Disturbance update Eq. (36)
% ============================
d_hat = d + Ts * beta2 * e0;

%% ============================
%  (5) Save states
% ============================
theta = theta_hat;
omega = omega_hat;
d     = d_hat;

end

== matlab function Simulacion_stepper_2024a/Subsystem1/Triggered Subsystem4/MATLAB Function ==
  data: Wm_ref input; Wm input; Vd output; Vq output; Id output; Iq output; Iq_ref output; X input; Theta_e input; Ts input; Vdc input; Imax input; Kp_w input; Ki_w input; Kp_d input; Ki_d input; Kp_q input; Ki_q input; Tl_tdm input; B input; Kt input; Ke input; L input; P input; R input
function [Vd,Vq,Id,Iq,Iq_ref] = PI_dq( ...
        Wm_ref, Wm, X, Theta_e, Ts, Vdc, Imax, ...
        Kp_w, Ki_w, Kp_d, Ki_d, Kp_q, Ki_q, ...
        Tl_tdm, B, Kt, Ke, L, P,R)

% ===== FIX DIMENSIONES: preasignar salidas (escalares) =====
Vd     = 0.0;
Vq     = 0.0;
Id     = 0.0;
Iq     = 0.0;
Iq_ref = 0.0;

persistent ek_w ek1_w u_w ...
           ek_d ek1_d u_d ...
           ek_q ek1_q u_q

    if isempty(ek_w)
        ek_w  = 0;   ek1_w = 0;   u_w  = 0;
        ek_d  = 0;   ek1_d = 0;   u_d  = 0;
        ek_q  = 0;   ek1_q = 0;   u_q  = 0;
       
    end

    %% ================== Transformada dq ==================
    Ia = X(1);
    Ib = X(2);

    C = cos(Theta_e);
    S = sin(Theta_e);

    Id =  Ia*C + Ib*S;
    Iq = -Ia*S + Ib*C;   % signo correcto

    %% ================== Control de velocidad ==================
    ek1_w = ek_w;
    ek_w  = Wm_ref - Wm;

    k1_w = Kp_w + Ki_w*Ts;
    k2_w = -Kp_w;

    du_w = k1_w*ek_w + k2_w*ek1_w;
    u_w  = u_w + du_w;

    % Feedforward de torque
    Iq_ff  = (Tl_tdm + B*Wm)/Kt;
    Iq_ref = Iq_ff + u_w;

    % Saturación de corriente (Iq_ref ≤ Imax)
    if abs(Iq_ref) > Imax
        Iq_ref = sign(Iq_ref)*Imax;
        % anti-windup del PI de velocidad
        u_w  = u_w - du_w;
        ek_w = ek1_w;
    end

    %% ================== Control PI de Iq ==================
    ek1_q = ek_q;
    ek_q  = Iq_ref - Iq;

    k1_q = Kp_q + Ki_q*Ts;
    k2_q = -Kp_q;

    du_q = k1_q*ek_q + k2_q*ek1_q;
    u_q  = u_q + du_q;

    %% ================== Control PI de Id (Id_ref = 0) ==================
    ek1_d = ek_d;
    ek_d  = -Id;

    k1_d = Kp_d + Ki_d*Ts;
    k2_d = -Kp_d;

    du_d = k1_d*ek_d + k2_d*ek1_d;
    u_d  = u_d + du_d;

    %% ================== DESACOPLES ==================
    We = P * Wm;   % velocidad eléctrica

    Vdec_d = Id*R -L * We * Iq;
    Vdec_q = Iq*R + Ke * Wm + L * We * Id;

    % Voltajes no saturados
    Vd = u_d + Vdec_d;
    Vq = u_q + Vdec_q;

    %% ================== SATURACIÓN CIRCULAR dq ==================
    Vnorm = sqrt(Vd^2 + Vq^2);

    if Vnorm > Vdc
        scale = Vdc / Vnorm;
        Vd_sat = Vd * scale;
        Vq_sat = Vq * scale;

        % Anti-windup PI de corriente
        u_d = Vd_sat - Vdec_d;
        u_q = Vq_sat - Vdec_q;

        Vd = Vd_sat;
        Vq = Vq_sat;
    end

end

== matlab function Simulacion_stepper_2024a/MATLAB Function6 ==
  data: u input; y output
function y = fcn(u)

y = wrap_2pi(u);

== matlab function Simulacion_stepper_2024a/Triggered Subsystem/MATLAB Function ==
  data: Wm_cmd input; Wm_ref output; Ts input; slope input; alpha_ref output
function [Wm_ref, alpha_ref] = ramp_generator(Wm_cmd, Ts, slope)

persistent Wm_ref_prev
if isempty(Wm_ref_prev)
    Wm_ref_prev = 0;
end

delta = Wm_cmd - Wm_ref_prev;

max_step = slope * Ts;

if delta > max_step
    delta = max_step;
elseif delta < -max_step
    delta = -max_step;
end

Wm_ref = Wm_ref_prev + delta;

% 🔥 aquí está la clave
alpha_ref = (Wm_ref - Wm_ref_prev)/Ts;

Wm_ref_prev = Wm_ref;

end

== matlab function Simulacion_stepper_2024a/Subsystem1/Triggered Subsystem2/MATLAB Function ==
  data: Wm_ref input; Wm input; Vd output; Vq output; Id output; Iq output; Iq_ref output; X input; Theta_e input; Ts input; Vdc input; Imax input; Kp_w input; Ki_w input; Kp_d input; Ki_d input; Kp_q input; Ki_q input; Tl_tdm input; B input; Kt input; Ke input; L input; P input; R input
function [Vd,Vq,Id,Iq,Iq_ref] = PI_dq( ...
        Wm_ref, Wm, X, Theta_e, Ts, Vdc, Imax, ...
        Kp_w, Ki_w, Kp_d, Ki_d, Kp_q, Ki_q, ...
        Tl_tdm, B, Kt, Ke, L, P,R)

persistent ek_w ek1_w u_w ...
           ek_d ek1_d u_d ...
           ek_q ek1_q u_q

    if isempty(ek_w)
        ek_w  = 0;   ek1_w = 0;   u_w  = 0;
        ek_d  = 0;   ek1_d = 0;   u_d  = 0;
        ek_q  = 0;   ek1_q = 0;   u_q  = 0;
    end

    %% ================== Transformada dq ==================
    Ia = X(1);
    Ib = X(2);

    C = cos(Theta_e);
    S = sin(Theta_e);

    Id =  Ia*C + Ib*S;
    Iq = -Ia*S + Ib*C;   % signo correcto

    %% ================== Control de velocidad ==================
    ek1_w = ek_w;
    ek_w  = Wm_ref - Wm;

    k1_w = Kp_w + Ki_w*Ts;
    k2_w = -Kp_w;

    du_w = k1_w*ek_w + k2_w*ek1_w;
    u_w  = u_w + du_w;

    % Feedforward de torque
    Iq_ff  = (Tl_tdm + B*Wm)/Kt;
    Iq_ref = Iq_ff + u_w;

    % Saturación de corriente (Iq_ref ≤ Imax)
    if abs(Iq_ref) > Imax
        Iq_ref = sign(Iq_ref)*Imax;
        % anti-windup del PI de velocidad
        u_w  = u_w - du_w;
        ek_w = ek1_w;
    end

    %% ================== Control PI de Iq ==================
    ek1_q = ek_q;
    ek_q  = Iq_ref - Iq;

    k1_q = Kp_q + Ki_q*Ts;
    k2_q = -Kp_q;

    du_q = k1_q*ek_q + k2_q*ek1_q;
    u_q  = u_q + du_q;

    %% ================== Control PI de Id (Id_ref = 0) ==================
    ek1_d = ek_d;
    ek_d  = -Id;

    k1_d = Kp_d + Ki_d*Ts;
    k2_d = -Kp_d;

    du_d = k1_d*ek_d + k2_d*ek1_d;
    u_d  = u_d + du_d;

    %% ================== DESACOPLES ==================
    We = P * Wm;   % velocidad eléctrica

    Vdec_d = Id*R -L * We * Iq;
    Vdec_q = Iq*R + Ke * Wm + L * We * Id;

    % Voltajes no saturados
    Vd = u_d + Vdec_d;
    Vq = u_q + Vdec_q;

    %% ================== SATURACIÓN CIRCULAR dq ==================
    Vnorm = sqrt(Vd^2 + Vq^2);

    if Vnorm > Vdc
        scale = Vdc / Vnorm;
        Vd_sat = Vd * scale;
        Vq_sat = Vq * scale;

        % Anti-windup PI de corriente
        u_d = Vd_sat - Vdec_d;
        u_q = Vq_sat - Vdec_q;

        Vd = Vd_sat;
        Vq = Vq_sat;
    end

end

== matlab function Simulacion_stepper_2024a/Triggered Subsystem5/MATLAB Function ==
  data: Wm input; Vd output; X input size=[2 1]; Theta_e input; Ts input; Vdc input; Kp_d input; Ki_d input; Kp_q input; Ki_q input; Psi input; Ld input; Lq input; P input; Vq output; Id_out output; Iq_out output; Iq_ref_req input; Valpha output; Vbetha output
function [Vd, Vq, Id_out, Iq_out,Valpha,Vbetha] = PI_dq_vectorial_fixed(Wm, X, Theta_e, Ts, Vdc, ...
                                           Kp_d, Ki_d, Kp_q, Ki_q, ...
                                           Psi, Ld, Lq, P, Iq_ref_req)
% Parámetros internos
I_max = sqrt(2); 
persistent v_int_d v_int_q Id_filt Iq_filt
if isempty(v_int_d)
    v_int_d = 0; 
    v_int_q = 0; 
    Id_filt = 0;
    Iq_filt = 0;
end

% 
%  fc_d = 1200; 
%  tau_d = 1/(2*pi*fc_d);
% alpha_d = tau_d/(tau_d + Ts); % Coeficiente del filtro
% 
%  fc_q = 600; 
%  tau_q = 1/(2*pi*fc_q);
% alpha_q = tau_q/(tau_q + Ts); % Coeficiente del filtro
%% 1. Transformada de Park
Ia = X(1); Ib = X(2);
cos_th = cos(Theta_e); sin_th = sin(Theta_e);



Id =  Ia * cos_th + Ib * sin_th;
Iq =  -Ia * sin_th + Ib * cos_th;

% % Aplicamos el filtro a la velocidad medida
 % Id_f = alpha_d * Id_filt + (1 - alpha_d) * Id;
 % Id_filt = Id_f; % Actualizamos el estado para la próxima iteración
 % 
 % % % Aplicamos el filtro a la velocidad medida
 % Iq_f = alpha_q * Iq_filt + (1 - alpha_q) * Iq;
 % Iq_filt = Iq_f; % Actualizamos el estado para la próxima iteración
%% 2. Referencias con Saturación Vectorial
Id_ref = 0; 
Iq_limit = sqrt(max(0, I_max^2 - Id_ref^2)); 
Iq_ref = max(-Iq_limit, min(Iq_limit, Iq_ref_req));

%% 3. Errores y Desacoples
err_d = Id_ref - Id;
err_q = Iq_ref - Iq;
We = P * Wm; 

% Términos de Desacople
V_cross_d = -We * Lq * Iq_ref; 
V_cross_q =  We * Ld * Id_ref + We * Psi; 

%% 4. Cálculo de Voltaje Base (PI + Feedforward)
Vd_pre = Kp_d * err_d + v_int_d + V_cross_d;
Vq_pre = Kp_q * err_q + v_int_q + V_cross_q;

%% 5. Protección de Corriente y Saturación de Voltaje
I_mag_real = sqrt(Id^2 + Iq^2);
limit_V = Vdc;

% Si la corriente real excede el límite de seguridad (1.2A)
if I_mag_real > 1.2
    limit_V = Vdc * (1.0 / I_mag_real);
end

% Saturación Circular de Voltaje
V_mag = sqrt(Vd_pre^2 + Vq_pre^2);

if V_mag > limit_V
    Vd = (Vd_pre / V_mag) * limit_V;
    Vq = (Vq_pre / V_mag) * limit_V;
    sat_active = true;
else
    Vd = Vd_pre;
    Vq = Vq_pre;
    sat_active = false;
end

%% 6. Anti-Windup (Clamping)
if ~sat_active || (sign(err_d) ~= sign(v_int_d))
    v_int_d = v_int_d + Ki_d * Ts * err_d;
end
if ~sat_active || (sign(err_q) ~= sign(v_int_q))
    v_int_q = v_int_q + Ki_q * Ts * err_q;
end

% Salidas de monitoreo
Id_out = Id; 
Iq_out = Iq;

%% 7. Transformada Inversa de Park (Salida a Marco Estacionario)
% Usamos el MISMO ángulo desfasado que en la entrada para mantener la coherencia
Valpha = Vd * cos(Theta_e) - Vq *sin(Theta_e);
Vbetha = Vd * sin(Theta_e) + Vq *cos(Theta_e);
end

== matlab function Simulacion_stepper_2024a/Triggered Subsystem6/MATLAB Function ==
  data: Wm_ref input; alpha_ref input; Wm input; Ts input; Kp_w input; Ki_w input; Tl_tdm input; B input; Kt input; theta_m input; Tdm input; J input; Phi input; Imax input; Iq_ref output; N_steps input; Iq_cogging output; Iq_PI output
function [Iq_ref,Iq_cogging,Iq_PI]  = PI_speed( ...
        Wm_ref,alpha_ref, Wm, Ts, ...
        Kp_w, Ki_w, ...
        Tl_tdm, B, Kt, theta_m, Tdm,J,Phi, ...
        Imax,N_steps)

% ================== Estados Persistentes ==================
% Añadimos Wm_filt para guardar el estado del filtro
persistent ek_w u_w Wm_filt
if isempty(u_w)
    u_w  = 0;
    ek_w = 0; 
    Wm_filt = Wm; % Inicializamos el filtro con el primer valor medido
end

% ================== Filtro Pasabajos (LPF) ==================
% Definimos la frecuencia de corte del filtro (fc). 
% Para un BW de velocidad de 20Hz, un fc de 50-100Hz es ideal.
%  fc = 150; 
%  tau = 1/(2*pi*fc);
% alpha = tau/(tau + Ts); % Coeficiente del filtro
% % 
% % % Aplicamos el filtro a la velocidad medida
%  Wm_f = alpha * Wm_filt + (1 - alpha) * Wm;
%  Wm_filt = Wm_f; % Actualizamos el estado para la próxima iteración

% ================== Feedforward (Modelo de la Planta) ==================
% Es mejor usar la velocidad filtrada para el término viscoso
Kff = 0.2;
Iq_ff = (J*alpha_ref +Tl_tdm + B*Wm_ref)/Kt;
Iq_cogging = Kff*(Tdm*sin(N_steps*theta_m + Phi)) / Kt;
% ================== PI incremental ==================
% El error ahora se calcula con la velocidad FILTRADA
ek_curr = Wm_ref - Wm;

k1_w = Kp_w + Ki_w*Ts;
k2_w = -Kp_w;

du_w = k1_w * ek_curr + k2_w * ek_w;
u_w  = u_w + du_w;

% La referencia final sin restricción de signo
Iq_ref_raw = Iq_ff + u_w + Iq_cogging;
Iq_ref = max(min(Iq_ref_raw, Imax), -Imax);

% ================== Saturación con Anti-Windup ==================
if abs(Iq_ref) > Imax
    Iq_ref = sign(Iq_ref) * Imax;
    u_w = u_w - du_w;
else
    ek_w = ek_curr;
end
Iq_PI = u_w;

end
